simulink subsystem "Controller"  (R2024a)
settings: Solver=VariableStepAuto  StartTime=0.0  StopTime=10.0  RelTol=1e-3
libraries: simulink_extras x6
settings Model: Creator=dylanfanner  LastModifiedBy=User

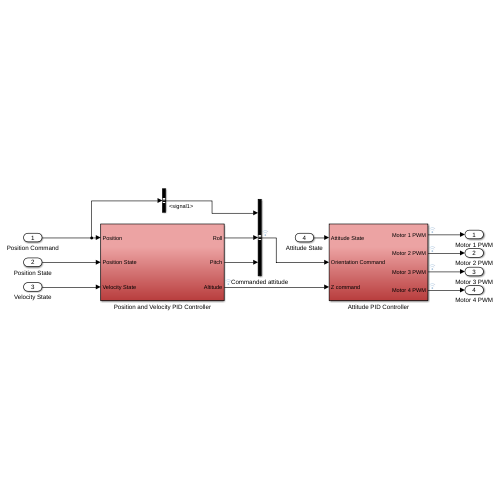
[thumbnail: Simulink's stored preview of the top-level diagram]
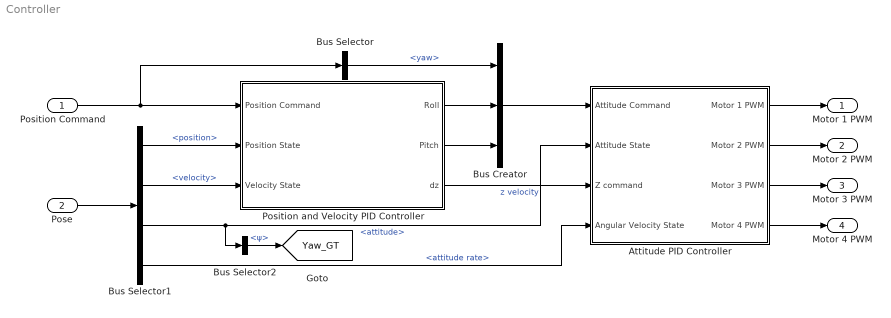
== system Controller ==
  Position Command : Inport
  Pose : Inport  Port=2
  Attitude PID Controller : Subsystem
  Bus Selector : BusSelector  OutputSignals=yaw
  Bus Selector1 : BusSelector  OutputSignals=Position State.position,Position State.velocity,Attitude State.attitude,Attitude State.attitude rate
  Bus Selector2 : BusSelector  OutputSignals=ψ
  Bus Creator : BusCreator  Inputs=3
  Position and Velocity PID Controller : Subsystem
  Motor 1 PWM : Outport
  Motor 2 PWM : Outport  Port=2
  Motor 3 PWM : Outport  Port=3
  Motor 4 PWM : Outport  Port=4
  tag scope: Yaw_GT=global
  wires:
  Position and Velocity PID Controller/2(Pitch) -> Bus Creator/3
  Attitude PID Controller/3(Motor 3 PWM) -> Motor 3 PWM/1
  Attitude PID Controller/2(Motor 2 PWM) -> Motor 2 PWM/1
  Position and Velocity PID Controller/1(Roll) -> Bus Creator/2
  Attitude PID Controller/1(Motor 1 PWM) -> Motor 1 PWM/1
  Position and Velocity PID Controller/3(dz) -> Attitude PID Controller/3(Z command)  "z velocity"
  Attitude PID Controller/4(Motor 4 PWM) -> Motor 4 PWM/1
  Position Command/1 -> Bus Selector/1, Position and Velocity PID Controller/1(Position Command)
  Bus Selector1/1 -> Position and Velocity PID Controller/2(Position State)  "<position>"
  Bus Selector1/2 -> Position and Velocity PID Controller/3(Velocity State)  "<velocity>"
  Bus Selector/1 -> Bus Creator/1  "<yaw>"
  Pose/1 -> Bus Selector1/1
  Bus Creator/1 -> Attitude PID Controller/1(Attitude Command)
  Bus Selector1/3 -> Attitude PID Controller/2(Attitude State), Bus Selector2/1  "<attitude>"
  Bus Selector1/4 -> Attitude PID Controller/4(Angular Velocity State)  "<attitude rate>"
  Bus Selector2/1 -> [Yaw_GT]  "<ψ>"

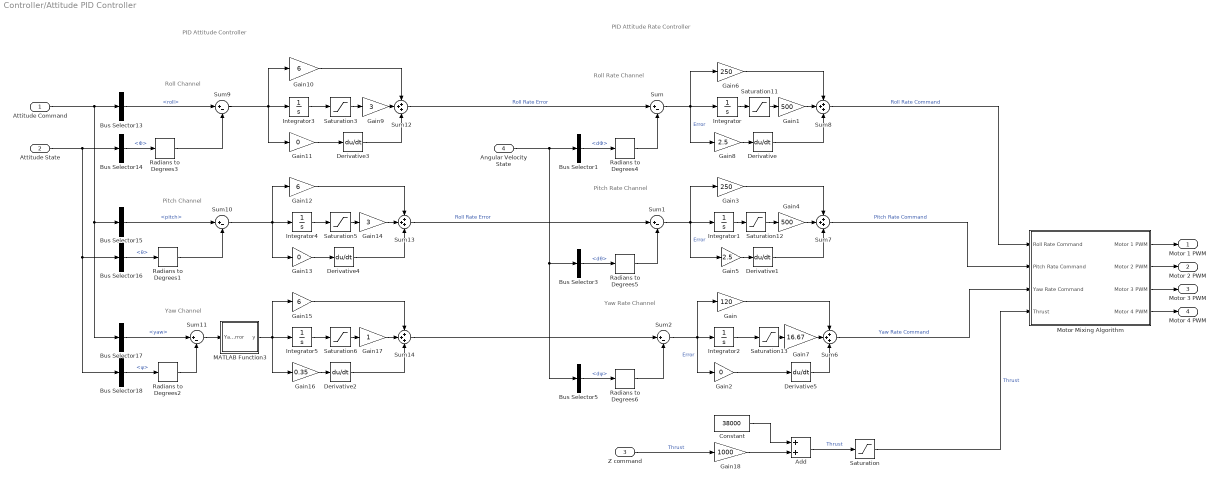
== system Controller/Attitude PID Controller ==
  note: Roll Channel
  note: PID Attitude Controller
  note: PID Attitude Rate Controller
  note: Pitch Channel
  note: Yaw Channel
  note: Roll Rate Channel
  note: Pitch Rate Channel
  note: Yaw Rate Channel
  Attitude Command : Inport
  Attitude State : Inport  Port=2
  Z command : Inport  Port=3
  Angular Velocity State : Inport  Port=4
  Add : Sum
  Bus Selector1 : BusSelector  OutputSignals=dΦ
  Bus Selector13 : BusSelector  OutputSignals=roll
  Bus Selector14 : BusSelector  OutputSignals=Φ
  Bus Selector15 : BusSelector  OutputSignals=pitch
  Bus Selector16 : BusSelector  OutputSignals=θ
  Bus Selector17 : BusSelector  OutputSignals=yaw
  Bus Selector18 : BusSelector  OutputSignals=ψ
  Bus Selector3 : BusSelector  OutputSignals=dθ
  Bus Selector5 : BusSelector  OutputSignals=dψ
  Constant : Constant  Value=38000
  Derivative{,1..5} (6 alike) : Derivative
  Gain : Gain  Gain=120
  Gain1 : Gain  Gain=500
  Gain10 : Gain  Gain=6
  Gain11 : Gain  Gain=0
  Gain12 : Gain  Gain=6
  Gain13 : Gain  Gain=0
  Gain14 : Gain  Gain=3
  Gain15 : Gain  Gain=6
  Gain16 : Gain  Gain=0.35
  Gain17 : Gain
  Gain18 : Gain  Gain=1000
  Gain2 : Gain  Gain=0
  Gain3 : Gain  Gain=250
  Gain4 : Gain  Gain=500
  Gain5 : Gain  Gain=2.5
  Gain6 : Gain  Gain=250
  Gain7 : Gain  Gain=16.67
  Gain8 : Gain  Gain=2.5
  Gain9 : Gain  Gain=3
  Integrator : Integrator  LimitOutput=on  UpperSaturationLimit=33.33  LowerSaturationLimit=-33.33
  Integrator1 : Integrator  LimitOutput=on  UpperSaturationLimit=33.33  LowerSaturationLimit=-33.3
  Integrator2 : Integrator  LimitOutput=on  UpperSaturationLimit=166.7  LowerSaturationLimit=-166.7
  Integrator3 : Integrator  LimitOutput=on  UpperSaturationLimit=20  LowerSaturationLimit=-20
  Integrator4 : Integrator  LimitOutput=on  UpperSaturationLimit=20  LowerSaturationLimit=-20
  Integrator5 : Integrator  LimitOutput=on  UpperSaturationLimit=360  LowerSaturationLimit=-360
  MATLAB Function3 : MATLAB Function  TreatAsAtomicUnit=on
  Motor Mixing Algorithm : Subsystem
  Radians to Degrees{1..6} (6 alike) : simulink_extras/Transformations/Radians to Degrees
  Saturation : Saturate  UpperLimit=65535  LowerLimit=20000
  Saturation11 : Saturate  UpperLimit=33.3  LowerLimit=-33.3
  Saturation12 : Saturate  UpperLimit=33.3  LowerLimit=-33.3
  Saturation13 : Saturate  UpperLimit=166.7  LowerLimit=-166.7
  Saturation3 : Saturate  UpperLimit=20  LowerLimit=-20
  Saturation5 : Saturate  UpperLimit=20  LowerLimit=-20
  Saturation6 : Saturate  UpperLimit=360  LowerLimit=-360
  Sum{,1..2,9..11} (6 alike) : Sum  Inputs=|+-
  Sum{6..8,12..14} (6 alike) : Sum  Inputs=+++
  Motor 1 PWM : Outport
  Motor 2 PWM : Outport  Port=2
  Motor 3 PWM : Outport  Port=3
  Motor 4 PWM : Outport  Port=4
  wires:
  Saturation/1 -> Motor Mixing Algorithm/4(Thrust)  "Thrust"
  Attitude State/1 -> Bus Selector18/1, Bus Selector16/1, Bus Selector14/1
  Z command/1 -> Gain18/1  "Thrust"
  Gain18/1 -> Add/2
  Bus Selector1/1 -> Radians to Degrees4/1  "<dΦ>"
  Bus Selector3/1 -> Radians to Degrees5/1  "<dθ>"
  Bus Selector5/1 -> Radians to Degrees6/1  "<dψ>"
  Angular Velocity State/1 -> Bus Selector1/1, Bus Selector3/1, Bus Selector5/1
  Gain/1 -> Sum6/1
  Gain3/1 -> Sum7/1
  Sum1/1 -> Integrator1/1, Gain5/1, Gain3/1  "Error"
  Gain6/1 -> Sum8/1
  Gain8/1 -> Derivative/1
  Sum/1 -> Integrator/1, Gain8/1, Gain6/1  "Error"
  Sum8/1 -> Motor Mixing Algorithm/1(Roll Rate Command)  "Roll Rate Command"
  Sum7/1 -> Motor Mixing Algorithm/2(Pitch Rate Command)  "Pitch Rate Command"
  Sum6/1 -> Motor Mixing Algorithm/3(Yaw Rate Command)  "Yaw Rate Command"
  Gain5/1 -> Derivative1/1
  Derivative1/1 -> Sum7/3
  Derivative/1 -> Sum8/3
  Gain1/1 -> Sum8/2
  Gain4/1 -> Sum7/2
  Sum2/1 -> Integrator2/1, Gain/1, Gain2/1  "Error"
  Gain7/1 -> Sum6/2
  Integrator/1 -> Saturation11/1
  Integrator1/1 -> Saturation12/1
  Integrator2/1 -> Saturation13/1
  Attitude Command/1 -> Bus Selector13/1, Bus Selector15/1, Bus Selector17/1
  Bus Selector14/1 -> Radians to Degrees3/1  "<Φ>"
  Bus Selector16/1 -> Radians to Degrees1/1  "<θ>"
  Bus Selector18/1 -> Radians to Degrees2/1  "<ψ>"
  Sum9/1 -> Integrator3/1, Gain11/1, Gain10/1
  Derivative3/1 -> Sum12/3
  Gain11/1 -> Derivative3/1
  Gain10/1 -> Sum12/1
  Gain9/1 -> Sum12/2
  Sum10/1 -> Gain13/1, Integrator4/1, Gain12/1
  Gain12/1 -> Sum13/1
  Gain14/1 -> Sum13/2
  Derivative4/1 -> Sum13/3
  Gain13/1 -> Derivative4/1
  Gain15/1 -> Sum14/1
  Gain17/1 -> Sum14/2
  Derivative2/1 -> Sum14/3
  Gain16/1 -> Derivative2/1
  Saturation11/1 -> Gain1/1
  Saturation12/1 -> Gain4/1
  Saturation13/1 -> Gain7/1
  Gain2/1 -> Derivative5/1
  Integrator3/1 -> Saturation3/1
  Integrator4/1 -> Saturation5/1
  Integrator5/1 -> Saturation6/1
  Saturation3/1 -> Gain9/1
  Saturation5/1 -> Gain14/1
  Saturation6/1 -> Gain17/1
  Radians to Degrees3/1 -> Sum9/2
  Radians to Degrees1/1 -> Sum10/2
  Radians to Degrees2/1 -> Sum11/2
  MATLAB Function3/1(y) -> Integrator5/1, Gain16/1, Gain15/1
  Sum11/1 -> MATLAB Function3/1(YawError)
  Derivative5/1 -> Sum6/3
  Radians to Degrees4/1 -> Sum/2
  Radians to Degrees5/1 -> Sum1/2
  Radians to Degrees6/1 -> Sum2/2
  Sum12/1 -> Sum/1  "Roll Rate Error"
  Sum13/1 -> Sum1/1  "Roll Rate Error"
  Sum14/1 -> Sum2/1
  Motor Mixing Algorithm/1(Motor 1 PWM) -> Motor 1 PWM/1
  Motor Mixing Algorithm/2(Motor 2 PWM) -> Motor 2 PWM/1
  Motor Mixing Algorithm/3(Motor 3 PWM) -> Motor 3 PWM/1
  Motor Mixing Algorithm/4(Motor 4 PWM) -> Motor 4 PWM/1
  Bus Selector13/1 -> Sum9/1  "<roll>"
  Bus Selector15/1 -> Sum10/1  "<pitch>"
  Bus Selector17/1 -> Sum11/1  "<yaw>"
  Add/1 -> Saturation/1  "Thrust"
  Constant/1 -> Add/1

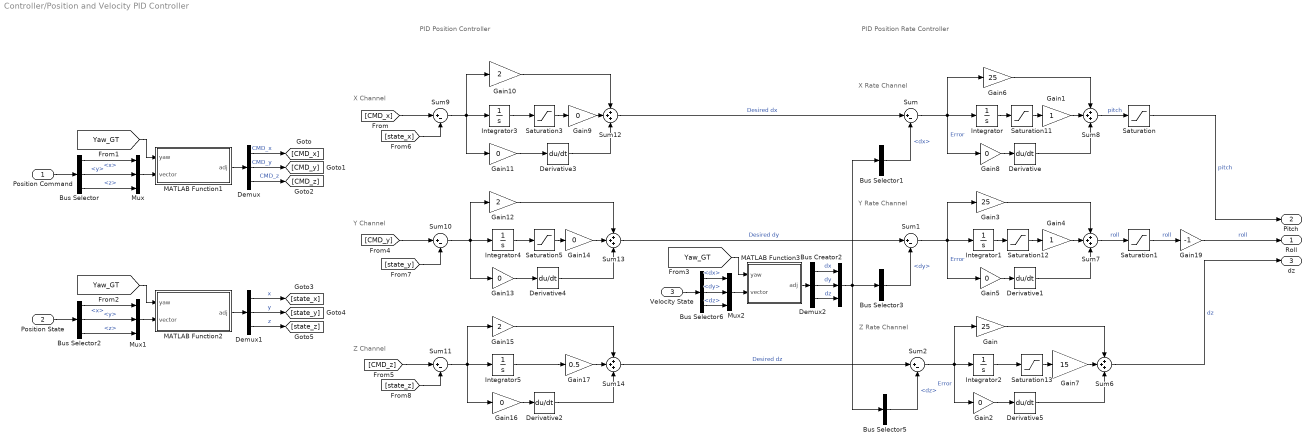
== system Controller/Position and Velocity PID Controller ==
  note: X Channel
  note: PID Position Controller
  note: PID Position Rate Controller
  note: Y Channel
  note: Z Channel
  note: X Rate Channel
  note: Y Rate Channel
  note: Z Rate Channel
  Position Command : Inport
  Position State : Inport  Port=2
  Velocity State : Inport  Port=3
  Bus Creator2 : BusCreator  Inputs=3
  Bus Selector : BusSelector  OutputSignals=x,y,z
  Bus Selector1 : BusSelector  OutputSignals=dx
  Bus Selector2 : BusSelector  OutputSignals=x,y,z
  Bus Selector3 : BusSelector  OutputSignals=dy
  Bus Selector5 : BusSelector  OutputSignals=dz
  Bus Selector6 : BusSelector  OutputSignals=dx,dy,dz
  Demux : Demux  Outputs=3
  Demux1 : Demux  Outputs=3
  Demux2 : Demux  Outputs=3
  Derivative{,1..5} (6 alike) : Derivative
  Gain : Gain  Gain=25
  Gain1 : Gain
  Gain10 : Gain  Gain=2
  Gain{2,5,8..9,11,13..14,16} (8 alike) : Gain  Gain=0
  Gain12 : Gain  Gain=2
  Gain15 : Gain  Gain=2
  Gain17 : Gain  Gain=0.5
  Gain19 : Gain  Gain=-1
  Gain3 : Gain  Gain=25
  Gain4 : Gain
  Gain6 : Gain  Gain=25
  Gain7 : Gain  Gain=15
  Integrator : Integrator  UpperSaturationLimit=33.33  LowerSaturationLimit=-33.33
  Integrator{1..5} (5 alike) : Integrator
  MATLAB Function1 : MATLAB Function  TreatAsAtomicUnit=on
  MATLAB Function2 : MATLAB Function  TreatAsAtomicUnit=on
  MATLAB Function3 : MATLAB Function  TreatAsAtomicUnit=on
  Mux : Mux  Inputs=3
  Mux1 : Mux  Inputs=3
  Mux2 : Mux  Inputs=3
  Saturation : Saturate  UpperLimit=20  LowerLimit=-20
  Saturation1 : Saturate  UpperLimit=20  LowerLimit=-20
  Saturation11 : Saturate  UpperLimit=1  LowerLimit=-1
  Saturation{3,5,12..13} (4 alike) : Saturate  UpperLimit=inf  LowerLimit=-inf
  Sum{,1..2,9..11} (6 alike) : Sum  Inputs=|+-
  Sum{6..8,12..14} (6 alike) : Sum  Inputs=+++
  Roll : Outport
  Pitch : Outport  Port=2
  dz : Outport  Port=3
  wires:
  [state_z] -> Sum11/2
  [state_y] -> Sum10/2
  [state_x] -> Sum9/2
  [CMD_z] -> Sum11/1
  [CMD_y] -> Sum10/1
  [CMD_x] -> Sum9/1
  Bus Selector6/3 -> Mux2/3  "<dz>"
  Bus Selector6/1 -> Mux2/1  "<dx>"
  Bus Selector6/2 -> Mux2/2  "<dy>"
  Velocity State/1 -> Bus Selector6/1
  Bus Creator2/1 -> Bus Selector3/1, Bus Selector5/1, Bus Selector1/1
  Demux2/2 -> Bus Creator2/2  "dy"
  Mux2/1 -> MATLAB Function3/2(vector)
  Demux2/3 -> Bus Creator2/3  "dz"
  Demux2/1 -> Bus Creator2/1  "dx"
  MATLAB Function3/1(adj) -> Demux2/1
  [Yaw_GT] -> MATLAB Function3/1(yaw)
  MATLAB Function2/1(adj) -> Demux1/1
  Position State/1 -> Bus Selector2/1
  Bus Selector2/2 -> Mux1/2  "<y>"
  Bus Selector2/1 -> Mux1/1  "<x>"
  Bus Selector2/3 -> Mux1/3  "<z>"
  Mux1/1 -> MATLAB Function2/2(vector)
  [Yaw_GT] -> MATLAB Function2/1(yaw)
  [Yaw_GT] -> MATLAB Function1/1(yaw)
  Mux/1 -> MATLAB Function1/2(vector)
  Bus Selector/3 -> Mux/3  "<z>"
  Bus Selector/1 -> Mux/1  "<x>"
  Bus Selector/2 -> Mux/2  "<y>"
  Demux1/1 -> [state_x]  "x"
  Demux1/2 -> [state_y]  "y"
  Demux1/3 -> [state_z]  "z"
  MATLAB Function1/1(adj) -> Demux/1
  Demux/3 -> [CMD_z]  "CMD_z"
  Demux/2 -> [CMD_y]  "CMD_y"
  Demux/1 -> [CMD_x]  "CMD_x"
  Position Command/1 -> Bus Selector/1
  Gain19/1 -> Roll/1  "roll"
  Saturation1/1 -> Gain19/1  "roll"
  Saturation/1 -> Pitch/1  "pitch"
  Sum6/1 -> dz/1  "dz"
  Sum7/1 -> Saturation1/1  "roll"
  Sum14/1 -> Sum2/1  "Desired dz"
  Bus Selector1/1 -> Sum/2  "<dx>"
  Bus Selector3/1 -> Sum1/2  "<dy>"
  Bus Selector5/1 -> Sum2/2  "<dz>"
  Gain/1 -> Sum6/1
  Gain3/1 -> Sum7/1
  Sum1/1 -> Integrator1/1, Gain5/1, Gain3/1  "Error"
  Gain6/1 -> Sum8/1
  Gain8/1 -> Derivative/1
  Sum/1 -> Integrator/1, Gain8/1, Gain6/1  "Error"
  Gain5/1 -> Derivative1/1
  Derivative1/1 -> Sum7/3
  Derivative/1 -> Sum8/3
  Gain1/1 -> Sum8/2
  Gain4/1 -> Sum7/2
  Sum2/1 -> Integrator2/1, Gain/1, Gain2/1  "Error"
  Gain7/1 -> Sum6/2
  Integrator/1 -> Saturation11/1
  Integrator1/1 -> Saturation12/1
  Integrator2/1 -> Saturation13/1
  Sum9/1 -> Integrator3/1, Gain11/1, Gain10/1
  Derivative3/1 -> Sum12/3
  Gain11/1 -> Derivative3/1
  Gain10/1 -> Sum12/1
  Gain9/1 -> Sum12/2
  Sum10/1 -> Gain13/1, Integrator4/1, Gain12/1
  Gain12/1 -> Sum13/1
  Gain14/1 -> Sum13/2
  Derivative4/1 -> Sum13/3
  Gain13/1 -> Derivative4/1
  Gain15/1 -> Sum14/1
  Gain17/1 -> Sum14/2
  Derivative2/1 -> Sum14/3
  Gain16/1 -> Derivative2/1
  Saturation11/1 -> Gain1/1
  Saturation12/1 -> Gain4/1
  Saturation13/1 -> Gain7/1
  Gain2/1 -> Derivative5/1
  Integrator3/1 -> Saturation3/1
  Integrator4/1 -> Saturation5/1
  Saturation3/1 -> Gain9/1
  Saturation5/1 -> Gain14/1
  Integrator5/1 -> Gain17/1
  Derivative5/1 -> Sum6/3
  Sum12/1 -> Sum/1  "Desired dx"
  Sum13/1 -> Sum1/1  "Desired dy"
  Sum8/1 -> Saturation/1  "pitch"
  Sum11/1 -> Integrator5/1, Gain15/1, Gain16/1

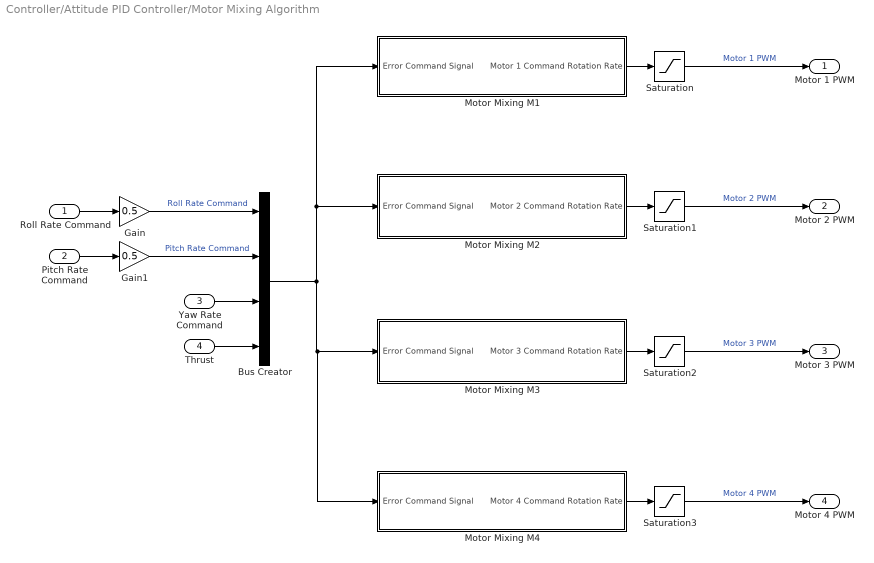
== system Controller/Attitude PID Controller/Motor Mixing Algorithm ==
  Roll Rate Command : Inport
  Pitch Rate Command : Inport  Port=2
  Yaw Rate Command : Inport  Port=3
  Thrust : Inport  Port=4
  Bus Creator : BusCreator  Inputs=4
  Gain : Gain  Gain=0.5
  Gain1 : Gain  Gain=0.5
  Motor Mixing M1 : Subsystem
  Motor Mixing M2 : Subsystem
  Motor Mixing M3 : Subsystem
  Motor Mixing M4 : Subsystem
  Saturation : Saturate  UpperLimit=65536  LowerLimit=-0  LinearizeAsGain=off  ZeroCross=off
  Saturation1 : Saturate  UpperLimit=65536  LowerLimit=-0  LinearizeAsGain=off  ZeroCross=off
  Saturation2 : Saturate  UpperLimit=65536  LowerLimit=0.  LinearizeAsGain=off  ZeroCross=off
  Saturation3 : Saturate  UpperLimit=65536  LowerLimit=0  LinearizeAsGain=off  ZeroCross=off
  Motor 1 PWM : Outport
  Motor 2 PWM : Outport  Port=2
  Motor 3 PWM : Outport  Port=3
  Motor 4 PWM : Outport  Port=4
  wires:
  Roll Rate Command/1 -> Gain/1
  Pitch Rate Command/1 -> Gain1/1
  Gain1/1 -> Bus Creator/2  "Pitch Rate Command"
  Gain/1 -> Bus Creator/1  "Roll Rate Command"
  Motor Mixing M3/1(Motor 3 Command Rotation Rate) -> Saturation2/1
  Motor Mixing M4/1(Motor 4 Command Rotation Rate) -> Saturation3/1
  Motor Mixing M2/1(Motor 2 Command Rotation Rate) -> Saturation1/1
  Motor Mixing M1/1(Motor 1 Command Rotation Rate) -> Saturation/1
  Yaw Rate Command/1 -> Bus Creator/3
  Thrust/1 -> Bus Creator/4
  Bus Creator/1 -> Motor Mixing M2/1(Error Command Signal), Motor Mixing M1/1(Error Command Signal), Motor Mixing M4/1(Error Command Signal), Motor Mixing M3/1(Error Command Signal)
  Saturation/1 -> Motor 1 PWM/1  "Motor 1 PWM"
  Saturation1/1 -> Motor 2 PWM/1  "Motor 2 PWM"
  Saturation2/1 -> Motor 3 PWM/1  "Motor 3 PWM"
  Saturation3/1 -> Motor 4 PWM/1  "Motor 4 PWM"

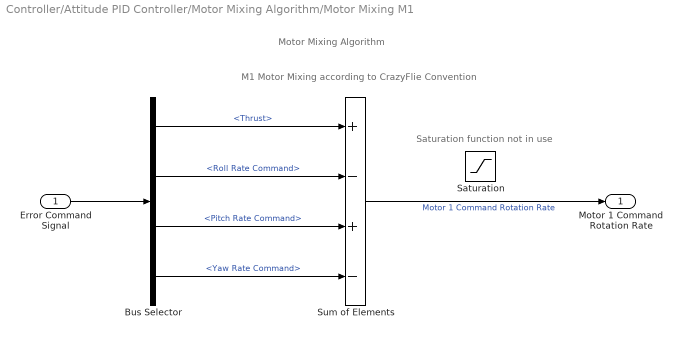
== system Controller/Attitude PID Controller/Motor Mixing Algorithm/Motor Mixing M1 ==
  note: Motor Mixing Algorithm
  note: M1 Motor Mixing according to CrazyFlie Convention
  note: Saturation function not in use
  Error Command Signal : Inport
  Bus Selector : BusSelector  OutputSignals=Thrust,Roll Rate Command,Pitch Rate Command,Yaw Rate Command
  Saturation : Saturate
  Sum of Elements : Sum  Inputs=+-+-
  Motor 1 Command Rotation Rate : Outport
  wires:
  Error Command Signal/1 -> Bus Selector/1
  Sum of Elements/1 -> Motor 1 Command Rotation Rate/1  "Motor 1 Command Rotation Rate"
  Bus Selector/3 -> Sum of Elements/3  "<Pitch Rate Command>"
  Bus Selector/4 -> Sum of Elements/4  "<Yaw Rate Command>"
  Bus Selector/2 -> Sum of Elements/2  "<Roll Rate Command>"
  Bus Selector/1 -> Sum of Elements/1  "<Thrust>"

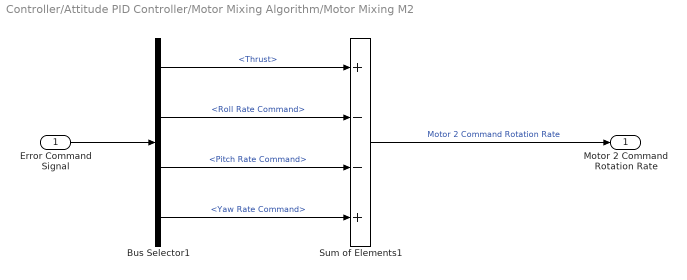
== system Controller/Attitude PID Controller/Motor Mixing Algorithm/Motor Mixing M2 ==
  Error Command Signal : Inport
  Bus Selector1 : BusSelector  OutputSignals=Thrust,Roll Rate Command,Pitch Rate Command,Yaw Rate Command
  Sum of Elements1 : Sum  Inputs=+--+
  Motor 2 Command Rotation Rate : Outport
  wires:
  Bus Selector1/4 -> Sum of Elements1/4  "<Yaw Rate Command>"
  Error Command Signal/1 -> Bus Selector1/1
  Bus Selector1/3 -> Sum of Elements1/3  "<Pitch Rate Command>"
  Bus Selector1/1 -> Sum of Elements1/1  "<Thrust>"
  Bus Selector1/2 -> Sum of Elements1/2  "<Roll Rate Command>"
  Sum of Elements1/1 -> Motor 2 Command Rotation Rate/1  "Motor 2 Command Rotation Rate"

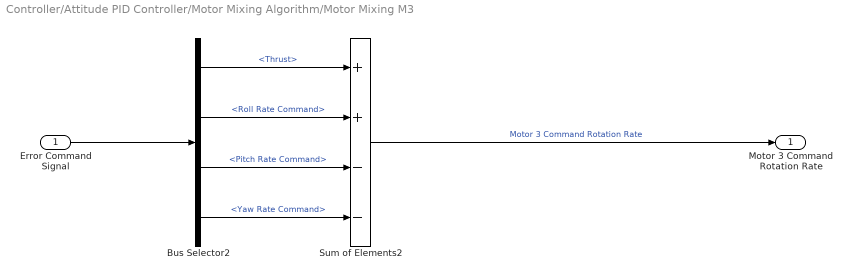
== system Controller/Attitude PID Controller/Motor Mixing Algorithm/Motor Mixing M3 ==
  Error Command Signal : Inport
  Bus Selector2 : BusSelector  OutputSignals=Thrust,Roll Rate Command,Pitch Rate Command,Yaw Rate Command
  Sum of Elements2 : Sum  Inputs=++--
  Motor 3 Command Rotation Rate : Outport
  wires:
  Bus Selector2/2 -> Sum of Elements2/2  "<Roll Rate Command>"
  Bus Selector2/1 -> Sum of Elements2/1  "<Thrust>"
  Error Command Signal/1 -> Bus Selector2/1
  Bus Selector2/4 -> Sum of Elements2/4  "<Yaw Rate Command>"
  Bus Selector2/3 -> Sum of Elements2/3  "<Pitch Rate Command>"
  Sum of Elements2/1 -> Motor 3 Command Rotation Rate/1  "Motor 3 Command Rotation Rate"

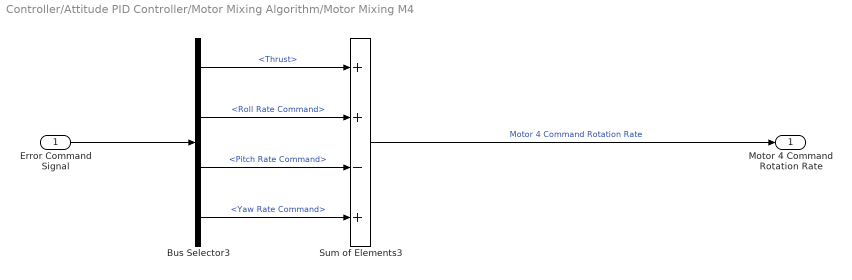
== system Controller/Attitude PID Controller/Motor Mixing Algorithm/Motor Mixing M4 ==
  Error Command Signal : Inport
  Bus Selector3 : BusSelector  OutputSignals=Thrust,Roll Rate Command,Pitch Rate Command,Yaw Rate Command
  Sum of Elements3 : Sum  Inputs=++-+
  Motor 4 Command Rotation Rate : Outport
  wires:
  Bus Selector3/4 -> Sum of Elements3/4  "<Yaw Rate Command>"
  Bus Selector3/2 -> Sum of Elements3/2  "<Roll Rate Command>"
  Sum of Elements3/1 -> Motor 4 Command Rotation Rate/1  "Motor 4 Command Rotation Rate"
  Bus Selector3/1 -> Sum of Elements3/1  "<Thrust>"
  Bus Selector3/3 -> Sum of Elements3/3  "<Pitch Rate Command>"
  Error Command Signal/1 -> Bus Selector3/1

== matlab function Controller/Position and Velocity PID Controller/MATLAB Function1 ==
  data: adj output; yaw input; vector input
function adj = fcn(yaw, vector)

adj = [cos(yaw) sin(yaw) 0;
        -sin(yaw) cos(yaw) 0;
         0 0 1] * vector;

== matlab function Controller/Position and Velocity PID Controller/MATLAB Function3 ==
  data: adj output; yaw input; vector input
function adj = fcn(yaw, vector)

adj = [cos(yaw) sin(yaw) 0;
        -sin(yaw) cos(yaw) 0;
         0 0 1] * vector;

== matlab function Controller/Attitude PID Controller/MATLAB Function3 ==
  data: YawError input; y output
function y = fcn(YawError)
YawError1=YawError;
if YawError>180
    YawError1=YawError-360;
end 
if YawError<-180
    YawError1=YawError+360;
end

y = YawError1;

== matlab function Controller/Position and Velocity PID Controller/MATLAB Function2 ==
  data: adj output; yaw input; vector input
function adj = fcn(yaw, vector)

adj = [cos(yaw) sin(yaw) 0;
        -sin(yaw) cos(yaw) 0;
         0 0 1] * vector;
